simulink model "generic_IVS"  (R2024a)
settings: Solver=FixedStepDiscrete  StartTime=0.0  StopTime=inf  FixedStep=0.001  RelTol=1e-3  EnableMultiTasking=on
undefined symbols (not defined in the file or in its folder): carLengthObs, dir, ego_Accel, ego_Speed, ego_X, ego_Y, ego_YAW, goalPosTol, goalYawTol, init_CurrentLaneInfo, init_DrivingMissionInfo, init_EgoVehicle, init_HybridAStarParam, init_MapData, init_ParkingMIssionInfo, is_Optimal_Path, isPathFound, LAD, lane_Coeff, lane_Idx, lane_waypoints, lane_waypoints_Length, lookAheadDistance, maxIter, missionState, obsRadius, parking_clear, parkingDestinationPos_X, parkingDestinationPos_Y, parkingDestinationYaw, parkingMapBoundary_X_Max, parkingMapBoundary_X_Min, parkingMapBoundary_Y_Max, parkingMapBoundary_Y_Min, parkingStartPos_X, parkingStartPos_Y, R_min, reversePenalty, Route1, route1_waypoint, Route2, route2_waypoint, Route3, route3_waypoint, Route_Parking, route_parking_waypoint, steerSet, stepSize, tollgateLaneNumber, vehicleRadius, velReference, xyResolution, y_LAD, y_lookAheadDistance, yawResolution, yawWeight
libraries: CarMaker4SL x48, simulink x1
(part 4 of 4)

== matlab function generic_IVS/CarMaker/Subsystem/Final Project/Scenario 1/Subsystem8/Global Waypoints To Local Transfomer ==
  settings: sampleTime=0.05
  data: waypointList input; current_lane_info input Bus: busCurrentLaneInfo; local_waypoints_ output size=[30 2]; ego_status input Bus: busEgoVehicle
function local_waypoints_ = global_to_local_waypoints(waypointList, current_lane_info, ego_status)

    num_waypoint = 15;
    vehicle_position = [ego_status.ego_X, ego_status.ego_Y];
    head = ego_status.ego_YAW;

    sub_waypointList = current_lane_info.lane_waypoints(1:current_lane_info.lane_waypoints_Length, :);

    if isempty(waypointList) || all(waypointList(:) == 0)
        waypoints = sub_waypointList;
    else
        waypoints = single(waypointList);
    end

    dx = waypoints(:,1) - vehicle_position(1);
    dy = waypoints(:,2) - vehicle_position(2);
    dist = dx.^2 + dy.^2;

    isNotForward = (dx*cos(head) + dy*sin(head)) < 0;
    dist(isNotForward) = inf;

    [~, idx_start] = min(dist);

    idx_end = idx_start + num_waypoint - 1;
    idx_end = min(idx_end, size(waypoints,1));
    selected = waypoints(idx_start:idx_end, :);

    L = size(selected,1);
    if L < num_waypoint
        selected = [selected; repmat(selected(end,:), num_waypoint-L, 1)];
    end

    R_inv = [ cos(head),  sin(head);
             -sin(head),  cos(head) ];

    delta = bsxfun(@minus, selected, vehicle_position);
    local_waypoints_ = (R_inv * delta')';

end

== matlab function generic_IVS/CarMaker/Subsystem/Final Project/Scenario 1/Subsystem8/MATLAB Function5 ==
  settings: sampleTime=0.001
  data: current_lane_info_out output Bus: busCurrentLaneInfo; current_lane_info_in input Bus: busCurrentLaneInfo; ego_status input
function current_lane_info_out = compute_lateral(current_lane_info_in, ego_status)
    
    current_lane_info_out = current_lane_info_in;
    poly_coeff = current_lane_info_in.lane_Coeff;

    lookahead_time = 1.7;
    velocity = ego_status.ego_Speed;
    x_lookahead = velocity * lookahead_time;
    degree = length(poly_coeff) - 1;

    y_ref = single(0.0);
    for i = 0:degree
        y_ref = y_ref + poly_coeff(i+1) * x_lookahead^i;
    end

    y_LAD = y_ref;
    LAD = sqrt(x_lookahead^2 + y_LAD^2);
    % disp('---lateral Node---')
    % disp(LAD)
    % disp(y_LAD)
    
    current_lane_info_out.lookAheadDistance = LAD;
    current_lane_info_out.y_lookAheadDistance = y_LAD;
    
end

== matlab function generic_IVS/CarMaker/Subsystem/Final Project/Scenario 1/Subsystem8/MATLAB Function6 ==
  settings: sampleTime=0.05
  data: local_waypoints input; current_lane_info_out output Bus: busCurrentLaneInfo; current_lane_info_in input Bus: busCurrentLaneInfo
function current_lane_info_out = fit_polynomial_to_waypoints(local_waypoints, current_lane_info_in)
    current_lane_info_out = fit_polynomial_to_waypoints_mfile(local_waypoints, current_lane_info_in);
end

function current_lane_info_out = fit_polynomial_to_waypoints_mfile(local_waypoints, current_lane_info_in)
    
    current_lane_info_out = current_lane_info_in;
    num_degree = 3;
    N = size(local_waypoints, 1);

    x = local_waypoints(:,1);
    b = local_waypoints(:,2);

    A = zeros(N, num_degree+1);
    for i = 0:num_degree
        A(:, i+1) = x.^i;
    end
    
    poly_coeff = pinv(A) * b;
    current_lane_info_out.lane_Coeff = poly_coeff;
    
    % disp('---polyfit Node---')
    % disp(current_lane_info_out.lane_Coeff)
    
end

== matlab function generic_IVS/CarMaker/Subsystem/Final Project/Scenario 1/Subsystem9/Lateral Control/MATLAB Function7 ==
  settings: updateMethod=DISCRETE  sampleTime=0.05
  data: current_lane_info input Bus: busCurrentLaneInfo; ego_status input Bus: busEgoVehicle; delta output
function delta  = lateral_stanley_controller_(current_lane_info, ego_status)
    
    k_h = 0.8;
    k_e = 0.4;

    heading_error = atan(current_lane_info.lane_Coeff(2));
    cross_track_error = current_lane_info.y_lookAheadDistance;
    V = ego_status.ego_Speed;
    
    heading_err_term     = k_h * heading_error;
    cross_track_err_term = atan(k_e * cross_track_error / V);

    delta = (heading_err_term + cross_track_err_term);
    
    V_thresh = 1;
    if abs(V) < V_thresh
        delta = 0;
        return;
    end

end

== matlab function generic_IVS/CarMaker/Subsystem/Final Project/Scenario 1/Subsystem9/Lateral Control/MATLAB Function8 ==
  settings: updateMethod=DISCRETE  sampleTime=0.05
  data: current_lane_info input Bus: busCurrentLaneInfo; delta output
function delta  = lateral_PP_controller_(current_lane_info)
    
    L = 2.9;  %wheelbase
    LAD = current_lane_info.lookAheadDistance;
    y_LAD = current_lane_info.y_lookAheadDistance;
    heading_error = current_lane_info.lane_Coeff(2);

    if LAD == 0
        disp('LAD = 0')
        delta = single(0.0);
        return
    end

    delta = 1.05*atan( 2 * L * y_LAD / (LAD^2) );

    % disp('---PP Node---')
    % disp(LAD)
    % disp(y_LAD)
    
end

== matlab function generic_IVS/CarMaker/Subsystem/Final Project/Scenario 1/get_adj_obstacles_info ==
  settings: sampleTime=0.05
  data: ego_status input; obstacles_info input [3..10]; adj output size=[8 10]; driving_mission_info input
function adj = get_adj_obstacles_info(ego_status, obstacles_info, driving_mission_info)
    % obstacles_info   : Nx matrix or struct (each obstacle row = one vehicle)
    %                    columns assumed: [X, Y, Vx, Vy, Ax, Ay, Yaw, Yawrate]

    % disp('--------')
    % disp(obstacles_info);
    % disp('--------')
    % disp('Vehicle_position')
    % disp(vehicle_position);
    % disp('--------')

    mission_state = driving_mission_info.missionState;
    if mission_state >= 3
        adj = zeros(3, 10);
        return;
    end
    
    dist_threshhold = 30.0;
    
    ego_x = ego_status.ego_X;
    ego_y = ego_status.ego_Y;

    X = obstacles_info(:,1);
    Y = obstacles_info(:,2);

    % 거리 계산
    dx = X - ego_x;
    dy = Y - ego_y;
    dist = dx.^2 + dy.^2;

    % threshold 안에 있는 인덱스
    idx = dist < dist_threshhold^2;

    % 필터링된 장애물 정보
    adj = obstacles_info(idx, :);
    
    % disp(idx);
    % if ~isempty(adj)
    %     disp('-----')
    %     disp(adj(1, :));
    % end
end

== matlab function generic_IVS/CarMaker/Subsystem/Final Project/Scenario 1/Set Velocity Reference ==
  settings: updateMethod=DISCRETE  sampleTime=0.05
  data: ego_status input Bus: busEgoVehicle; driving_mission_info_out output Bus: busDrivingMissionInfo; driving_mission_info_in input
function driving_mission_info_out = set_velocity_ref(ego_status, driving_mission_info_in)
    
    driving_mission_info_out = driving_mission_info_in;
    target_velocity = driving_mission_info_in.velReference;
    mission_state = driving_mission_info_in.missionState;

    ego_X = ego_status.ego_X;
    ego_Y = ego_status.ego_Y;

    lane_section_idx = get_lane_section_idx(ego_X, ego_Y);

    if lane_section_idx == 0
        mission_state = uint8(4);
    end

    if lane_section_idx == 1
        target_velocity = single(55/3.6);
    elseif lane_section_idx == 3 || lane_section_idx == 6
        target_velocity = single(45/3.6);
    elseif lane_section_idx == 4
        target_velocity = single(50/3.6);
    elseif lane_section_idx == 5
        target_velocity = single(55/3.6);
    elseif lane_section_idx == 7
        target_velocity = single(50/3.6);
    
    % 직선도로
    elseif lane_section_idx == 8
        target_velocity = single(65/3.6);
    end

    
    if mission_state == 2
        target_velocity = single(30/3.6);

    elseif mission_state == 3
        target_velocity = single(20/3.6);

        if lane_section_idx == 9
            target_velocity = single(8/3.6);
        end

    elseif mission_state == 4
        target_velocity = single(0.0);
    end

    driving_mission_info_out.velReference = target_velocity;

end

function lane_section_idx = get_lane_section_idx(ego_x, ego_y)
    % 섹션 1
    section1_x = [-50.6, -50.6, -99.25, -154, -168.38, -169];
    section1_y = [27,11.6, -18.32, -46.77, -39.43,27]; 
    
    % 섹션 2
    section2_x = [-168.38, -154, -151, -166.95, -178.59, -187];
    section2_y = [-39.43, -46.77, -69.31, -85.52, -85.52, -55];
    
    % 섹션 3
    section3_x = [-178.59, -166.95, -104, -36.24, -25.19, -25.19, -178.59];
    section3_y = [-85.52, -85.52, -85.52, -110.78, -115.02, -172, -172];
    
    % 섹션 4
    section4_x = [-36.24, -25.19, 3, 4.57, 0.49, -32];
    section4_y = [-110.78, -115.02, -113, -87.46, -76, -77];
    
    % 섹션 5
    section5_x = [ 0.49, 4.57, 41, 81.24, 81.24, 33];
    section5_y = [-76, -87.46, -85, -78.92, -63.15, -55];
    
    % 섹션 6
    section6_x = [81.24, 81.24, 111.99, 124.34, 124.4];
    section6_y = [-78.92, -63.15, -38.14, -38.14, -78.92];
    
    % 섹션 7
    section7_x = [60, 60, 111.99, 124.34, 124.34];
    section7_y = [27, 11.6, -38.14, -38.14, 27];
    
    % 섹션 8 직선도로
    section8_x = [-50.6, -50.6, 60, 60];
    section8_y = [27, 11.6, 11.6, 27];
    
    % 섹션 9 주차장 입구
    section9_x = [-9.8,5.5,-9.8,5.5];
    section9_y = [11.6, 11.6,-45,-45];

    polygon_list = {
        section1_x,  section1_y;
        section2_x,  section2_y;
        section3_x,  section3_y;
        section4_x,  section4_y;
        section5_x,  section5_y;
        section6_x,  section6_y;
        section7_x,  section7_y;
        section8_x,  section8_y;
        section9_x,  section9_y;
    };
    
    lane_section_idx = uint8(0);

    for i = 1:size(polygon_list,1)
        px = polygon_list{i,1};
        py = polygon_list{i,2};

        inside = inpolygon(ego_x, ego_y, px, py);

        if inside
            lane_section_idx = uint8(i);
            return;
        end
    end

end

== matlab function generic_IVS/CarMaker/Subsystem/Final Project/Scenario 1/MATLAB Function ==
  data: parking_mission_info input Bus: busParkingMissionInfo; path output size=[20000 4]; obstacles input; param input Bus: busHybridAStarParam
function path = hybridAstar_planner(parking_mission_info, obstacles, param)
    
    persistent initialized
    persistent cached_path
    persistent cached_len

    MAX_PATH = 20000;
    if isempty(initialized)
        initialized = false;
        cached_path = zeros(MAX_PATH, 4, 'single');
        cached_len  = uint16(0);
    end

    if initialized
        path = cached_path(1:cached_len, :);
        return;
    end
    x_min = parking_mission_info.parkingMapBoundary_X_Min;
    x_max = parking_mission_info.parkingMapBoundary_X_Max;
    y_min = parking_mission_info.parkingMapBoundary_Y_Min;
    y_max = parking_mission_info.parkingMapBoundary_Y_Max;
    
    space = [x_min, x_max, y_min, y_max];

    start_X   = parking_mission_info.parkingStartPos_X;
    start_Y   = parking_mission_info.parkingStartPos_Y;
    start_YAW = 0;

    obstacles = obstacles(:,1:3);
    
    goal_X   = parking_mission_info.parkingDestinationPos_X;
    goal_Y   = parking_mission_info.parkingDestinationPos_Y;
    goal_YAW = parking_mission_info.parkingDestinationYaw;

    goal = [goal_X, goal_Y, goal_YAW];

    p = param;

    nx = single(floor((x_max - x_min) / p.xyResolution) + 1);
    ny = single(floor((y_max - y_min) / p.xyResolution) + 1);
    nyaw = single(floor(2*pi / p.yawResolution) + 1);
    
    costList    = inf(nx, ny, nyaw);
    nodeIdList  = zeros(nx, ny, nyaw);
    closedList  = false(nx, ny, nyaw);
    
    MAX_NODES   = 20000;
    MAX_OPENSET = 20000;
    MAX_CHILDREN = 6;

    nodeTemplate = struct('x',single(0), 'y',single(0), 'yaw',single(0),...
                          'g',single(0), 'h',single(0), 'f',single(0),...
                          'dir',single(1), 'parent',int32(0),...
                          'ix',single(0), 'iy',single(0), 'iyaw',single(0));

    nodes = repmat(nodeTemplate, MAX_NODES, 1);
    nodeCount = 1;

    [ix,iy,iyaw] = world2grid(start_X, start_Y, start_YAW, ...
                              x_min, y_min, p.xyResolution, p.yawResolution);

    nodes(1).x    = start_X;
    nodes(1).y    = start_Y;
    nodes(1).yaw  = wrapToPi_local(start_YAW);
    nodes(1).g    = single(0.0);
    nodes(1).h    = heuristic_cost(start_X, start_Y, start_YAW, goal, p);
    nodes(1).f    = nodes(1).g + nodes(1).h;
    nodes(1).dir  = single(1.0);
    nodes(1).parent = int32(0);
    nodes(1).ix   = ix;
    nodes(1).iy   = iy;
    nodes(1).iyaw = iyaw;

    costList(ix,iy,iyaw)   = 0;
    nodeIdList(ix,iy,iyaw) = 1;

    openSet     = zeros(MAX_OPENSET, 1, 'int32');
    openCount   = 1;
    openSet(1)  = 1;

    success = false;
    goalId  = int32(-1);

    iter = 0;
    while (openCount > 0) && (iter < p.maxIter)
        iter = iter + 1;

        bestIdx = 1;
        bestId  = openSet(1);
        bestF   = nodes(bestId).f;
        
        for i = 2:openCount
            nid = openSet(i);
            if nodes(nid).f < bestF
                bestF = nodes(nid).f;
                bestIdx = i;
                bestId  = nid;
            end
        end
        
        curId = bestId;
        openSet(bestIdx) = openSet(openCount);  % 마지막 원소와 교체
        openCount = openCount - 1;

        curNode = nodes(curId);
        if closedList(curNode.ix, curNode.iy, curNode.iyaw)
            continue;
        end
        closedList(curNode.ix, curNode.iy, curNode.iyaw) = true;

        if isGoalReached(curNode, goal, p)
            success = true;
            goalId  = int32(curId);
            break;
        end

        children = CreateNode(curNode, p);

        for k = 1:numel(children)
            child = children(k);

            if child.x < x_min || child.x > x_max || ...
               child.y < y_min || child.y > y_max
                continue;
            end

            if checkCollisionMotion(curNode, child, obstacles, space, p)
                continue;
            end

            [ix_c,iy_c,iyaw_c] = world2grid(child.x, child.y, child.yaw, ...
                                            x_min, y_min, ...
                                            p.xyResolution, p.yawResolution);

            if closedList(ix_c,iy_c,iyaw_c)
                continue;
            end

            g_new = curNode.g + child.cost;

            if g_new < costList(ix_c,iy_c,iyaw_c)
                childNode = nodeTemplate;
                childNode.x    = child.x;
                childNode.y    = child.y;
                childNode.yaw  = wrapToPi_local(child.yaw);
                childNode.g    = g_new;
                childNode.h    = heuristic_cost(childNode.x, childNode.y, childNode.yaw, goal, p);
                childNode.f    = childNode.g + childNode.h;
                childNode.dir  = child.dir;
                childNode.parent = curId;
                childNode.ix   = ix_c;
                childNode.iy   = iy_c;
                childNode.iyaw = iyaw_c;

                if nodeIdList(ix_c,iy_c,iyaw_c) == 0
                    nodeCount = nodeCount + 1;
                    if nodeCount > MAX_NODES
                        continue;
                    end

                    nodes(nodeCount) = childNode;
                    newId = nodeCount;
                else
                    newId = nodeIdList(ix_c,iy_c,iyaw_c);
                    nodes(newId) = childNode;
                end

                costList(ix_c,iy_c,iyaw_c)   = g_new;
                nodeIdList(ix_c,iy_c,iyaw_c) = newId;
                
                if openCount < MAX_OPENSET
                    openCount = openCount + 1;
                    openSet(openCount) = newId;
                else
                end

            end
        end
    end

    if ~success
        path = zeros(1,4,'single');
        if ~initialized
            visualize_hybridAstar_internal(path, obstacles, [start_X start_Y], [goal_X goal_Y], p);
            initialized = true;
        end
        disp('no path')
        return;
    end

    path = backtrackPath(nodes, goalId, MAX_NODES);
    disp('find path')
    
    valid = (path(:,1) ~= 0) | (path(:,2) ~= 0) | (path(:,3) ~= 0);
    path = path(valid, :);

    k = size(path,1);
    cached_path(1:k, :) = path;
    cached_len = uint16(k);
    initialized = true;

    visualize_hybridAstar_internal(path, obstacles, [start_X start_Y], [goal_X goal_Y], p);
end



function ang = wrapToPi_local(ang)
    ang = single(mod(ang + pi, 2*pi) - pi);
end

% 양자화 때리는거
function [ix, iy, iyaw] = world2grid(x, y, yaw, x_min, y_min, res_xy, res_yaw)
    ix = floor((x - x_min) / res_xy) + 1;
    iy = floor((y - y_min) / res_xy) + 1;
    yaw = wrapToPi_local(yaw);
    iyaw = floor((yaw + pi) / res_yaw) + 1;
end

% 도착했는지 검사
function flag = isGoalReached(node, goal, p)
    dx = goal(1) - node.x;
    dy = goal(2) - node.y;
    dist = sqrt(dx^2 + dy^2);

    dyaw = abs(wrapToPi_local(goal(3) - node.yaw));
    flag = (dist < p.goalPosTol) && (dyaw < p.goalYawTol);
end

% 자식낳기
function children = CreateNode(node, p)

    R = p.R_min;
    kappa_max = 1.0 / R;
    ds = p.stepSize;

    steeringSet = p.steerSet * kappa_max;
    dirSet = [1, -1];

    MAX_CHILDREN = 6;
    children = repmat(struct('x',single(0), 'y',single(0), 'yaw',single(0), ...
                             'dir',single(0), 'cost',single(0)), single(MAX_CHILDREN), single(1));
    childCount = 0;

    for i = 1:length(steeringSet)

        kappa = steeringSet(i);
        for d = 1:length(dirSet)
            dir = dirSet(d);
            s   = dir * ds;

            [xn, yn, yawn] = BicycleKinematic(node.x, node.y, node.yaw, kappa, s);

            % cost: 경로 길이 + 후진 패널티
            cost = abs(ds);
            if dir < 0
                cost = cost * p.reversePenalty;
            end

            childCount = childCount + 1;
            children(childCount).x    = xn;
            children(childCount).y    = yn;
            children(childCount).yaw  = yawn;
            children(childCount).dir  = single(dir);
            children(childCount).cost = cost;
        end
    end
end

% Bicycle 모델
function [x_new, y_new, yaw_new] = BicycleKinematic(x, y, yaw, kappa, s)
    if abs(kappa) < 1e-6

        x_new   = x + s * cos(yaw);
        y_new   = y + s * sin(yaw);
        yaw_new = yaw;
    else

        R = 1.0 / kappa;
        yaw_new = yaw + kappa * s;
        x_new = x + R * (sin(yaw_new) - sin(yaw));
        y_new = y - R * (cos(yaw_new) - cos(yaw));
    end
    yaw_new = wrapToPi_local(yaw_new);
end

% 중간 샘플 몇 개 찍어서 충돌 체크 할거임
function flag = checkCollisionMotion(n1, n2, obstacles, space, p)
    
    nSamples = 5;
    flag = false;

    kappa_est = curvatureFromNodes(n1, n2, p);

    for i = 0:nSamples
        t  = i / nSamples;
        s  = t * p.stepSize * sign(n2.dir); % 방향 고려
        [x_s, y_s, ~] = BicycleKinematic(n1.x, n1.y, n1.yaw, ...
                                           kappa_est, s);

        if checkCollisionPoint(x_s, y_s, obstacles, space, p)
            flag = true;
            return;
        end
    end
end

function flag = checkCollisionPoint(x, y, obstacles, space, p)
    % World boundary
    if x < space(1) || x > space(2) || ...
       y < space(3) || y > space(4)
        flag = true;
        return;
    end

    % 장애물: 뒷대가리 기준 + heading → 차량 길이 따라 원 2개 배치
    L = p.carLengthObs;
    
    d1 = L * 0.3;    % 뒤쪽 쪽
    d2 = L * 0.8;    % 앞쪽 쪽

    effR2 = (p.obsRadius + p.vehicleRadius)^2;

    for i = 1:size(obstacles,1)
        xr = obstacles(i,1);
        yr = obstacles(i,2);
        hdg = obstacles(i,3);

        % 두 개 서클의 중심
        x1 = xr + d1*cos(hdg);
        y1 = yr + d1*sin(hdg);
        x2 = xr + d2*cos(hdg);
        y2 = yr + d2*sin(hdg);

        dx1 = x - x1; dy1 = y - y1;
        dx2 = x - x2; dy2 = y - y2;

        if (dx1*dx1 + dy1*dy1 < effR2) || (dx2*dx2 + dy2*dy2 < effR2)
            flag = true;
            return;
        end
    end

    flag = false;
end

function kappa = curvatureFromNodes(n1, n2, p)
    % n1→n2 κ 추정 (대충 yaw 변화로 계산)
    ds = p.stepSize;
    dyaw = wrapToPi_local(n2.yaw - n1.yaw);
    if abs(ds) < 1e-6
        kappa = single(0);
    else
        kappa = single(dyaw / (ds * sign(n2.dir)));
    end
end

function h = heuristic_cost(x, y, yaw, goal, p)
    dx = goal(1) - x;
    dy = goal(2) - y;
    dist = sqrt(dx^2 + dy^2);

    dyaw = abs(wrapToPi_local(goal(3) - yaw));
    h = dist + p.yawWeight * dyaw;
end

function path = backtrackPath(nodes, goalId, MAX_PATH)
    path = zeros(MAX_PATH, 4, 'single');

    idx = goalId;
    k = 0;
    
    % 뒤에서부터 채우고 뒤집음
    while (idx ~= 0) && (k < MAX_PATH)
        n = nodes(idx);
        k = k + 1;
        path(k, :) = [n.x, n.y, n.yaw, n.dir];
        idx = n.parent;
    end

    if k > 1
        % start→goal 순서로 뒤집기
        path(1:k, :) = flipud(path(1:k, :));
    end
end

% 시각화 (한번만 함)
function visualize_hybridAstar_internal(path, obstacles, startXY, goalXY, p)

    figure; hold on; axis equal; grid on;
    xlabel('X'); ylabel('Y');
    title('Hybrid A* Path');

    for i = 1:size(obstacles,1)
        drawObstacleCarDual(obstacles(i,1), obstacles(i,2), obstacles(i,3), p);
    end

    % Start & Goal
    plot(startXY(1), startXY(2), 'go', 'MarkerFaceColor','g','MarkerSize',10);
    plot(goalXY(1),  goalXY(2),  'ro', 'MarkerFaceColor','r','MarkerSize',10);

    % Path
    xs = path(:,1); ys = path(:,2); dirs = path(:,4);
    valid = xs ~= 0;
    xs = xs(valid); ys = ys(valid); dirs = dirs(valid);

    for i = 1:length(xs)-1
        if dirs(i) > 0
            plot(xs(i:i+1), ys(i:i+1), 'b-', 'LineWidth', 2);
        else
            plot(xs(i:i+1), ys(i:i+1), 'r-', 'LineWidth', 2);
        end
    end

    hold off;
end


function h = drawCircle(x, y, r, color)
    th = linspace(0, 2*pi, 40);
    xc = x + r*cos(th);
    yc = y + r*sin(th);
    h = fill(xc, yc, color, 'FaceAlpha', 0.3, 'EdgeColor', color);
end

function drawObstacleCarDual(xr, yr, hdg_deg, p)
    L   = p.carLengthObs;
    hdg = hdg_deg;

    d1 = L * 0.3;
    d2 = L * 0.8;

    x1 = xr + d1*cos(hdg);
    y1 = yr + d1*sin(hdg);
    x2 = xr + d2*cos(hdg);
    y2 = yr + d2*sin(hdg);

    drawCircle(x1, y1, p.obsRadius, [0.7 0.2 0.2]);
    drawCircle(x2, y2, p.obsRadius, [0.7 0.2 0.2]);
end

== matlab function generic_IVS/CarMaker/Subsystem/Final Project/Scenario 1/Global Waypoints To Local Transfomer ==
  settings: sampleTime=0.05
  data: mission_state input; parking_mission_info_in input Bus: busParkingMissionInfo; parking_mission_info_out output Bus: busParkingMissionInfo; waypoints input; ego_status input Bus: busEgoVehicle
function parking_mission_info_out  = global_to_local_path_manager(mission_state, parking_mission_info_in, waypoints, ego_status)
    
    parking_mission_info_out = parking_mission_info_in;
    
    if mission_state ~= 4
        return;
    end

    goalX = parking_mission_info_in.parkingDestinationPos_X;
    goalY = parking_mission_info_in.parkingDestinationPos_Y;
    ego_X = ego_status.ego_X;
    ego_Y = ego_status.ego_Y;

    dx_goal = ego_X - goalX;
    dy_goal = ego_Y - goalY;
    dist_goal = sqrt(dx_goal^2 + dy_goal^2);

    if dist_goal < 1.0
        parking_mission_info_out.parking_clear = uint8(1);
        parking_mission_info_out.LAD = single(0.01);
        parking_mission_info_out.y_LAD = single(0.0);
        disp("Parking!")
        return;
    end
    
    if size(waypoints,1) == 1 && (max(abs(waypoints(:))) == 0)
        parking_mission_info_out.isPathFound = uint8(0);
        parking_mission_info_out.LAD = single(0.0);
        parking_mission_info_out.y_LAD = single(0.0);
        return;
    else
        parking_mission_info_out.isPathFound = uint8(1);
    end
    num_waypoint = 5;

    vehicle_position = [ego_X, ego_Y];
    head = ego_status.ego_YAW;

    dx = waypoints(:,1) - vehicle_position(1);
    dy = waypoints(:,2) - vehicle_position(2);
    dist = dx.^2 + dy.^2;

    % isNotForward = (dx*cos(head) + dy*sin(head)) < 0;
    % dist(isNotForward) = inf;

    [minDist, idx_start] = min(dist);
    
    % disp('---minDist---')
    % disp(minDist)
    % if minDist > 3.0
    %     parking_mission_info_out.LAD = single(0.0);
    %     parking_mission_info_out.y_LAD = single(0.0);
    %     parking_mission_info_out.dir = int8(-1);
    %    return;
    % end

    idx_end = idx_start + num_waypoint - 1;
    idx_end = min(idx_end, size(waypoints,1));
    selected = waypoints(idx_start:idx_end, :);

    L = size(selected,1);
    if L < num_waypoint
        selected = [selected; repmat(selected(end,:), num_waypoint-L, 1)];
    end

    R_inv = [ cos(head),  sin(head);
             -sin(head),  cos(head) ];
    
    selected_xy = selected(:,1:2);
    delta = bsxfun(@minus, selected_xy, vehicle_position);
    local_waypoints_ = (R_inv * delta')';

    poly_coeff  = fit_polynomial_to_waypoints_mfile(local_waypoints_);
    [y_LAD, LAD] = compute_lateral(poly_coeff);
    dir = int8(waypoints(idx_start,4));

    % disp(size(waypoints(:,1)))
    % disp(idx_start)
    % disp(waypoints(idx_start, :))
    
    parking_mission_info_out.LAD = LAD;
    parking_mission_info_out.y_LAD = y_LAD;
    parking_mission_info_out.dir = dir;

end

function  poly_coeff  = fit_polynomial_to_waypoints_mfile(local_waypoints)

    num_degree = 3;
    N = size(local_waypoints, 1);

    x = local_waypoints(:,1);
    b = local_waypoints(:,2);

    A = zeros(N, num_degree+1);
    for i = 0:num_degree
        A(:, i+1) = x.^i;
    end
    
    poly_coeff = pinv(A) * b;
    
end

function [y_LAD, LAD] = compute_lateral(poly_coeff)

    x_lookahead = 2.9 + 0.6;
    degree = length(poly_coeff) - 1;

    y_ref = single(0.0);
    for i = 0:degree
        y_ref = y_ref + poly_coeff(i+1) * x_lookahead^i;
    end

    y_LAD = single(y_ref);
    LAD = single(sqrt(x_lookahead^2 + y_LAD^2));
    
end

== stateflow chart generic_IVS/CarMaker/Subsystem/Final Project/Scenario 1/Subsystem7/Chart3 ==
  state driving
    mission=1;
  state tollgate
    mission=2;
  state parking_entry
    mission=3;
  state parking
    mission=4;
  (default) -> driving
  driving -> tollgate [order 1] : [flag_2==1]
  tollgate -> driving : [flag_2==0]
  driving -> parking_entry [order 2] : [flag_3==1]
  parking_entry -> parking : [flag_4==1]
  data: flag_2 input; flag_3 input; mission output; flag_4 input

== matlab function generic_IVS/CarMaker/Subsystem/Final Project/Scenario 1/Subsystem6/MATLAB Function9 ==
  data: ego_status input; tollgate_pass_mode output
function tollgate_pass_mode = check_tollgate(ego_status)
% CHECK_TOLLGATE_ZONE: 에고 차량이 톨게이트 영역 내에 있는지 확인하여 플래그를 반환합니다.
%
% 입력:
%   ego_global_x: 에고 차량의 현재 글로벌 X 좌표 (float)
%   ego_global_y: 에고 차량의 현재 글로벌 Y 좌표 (float)


% 출력:
%   tollgate_pass_mode: 0 (영역 밖) 또는 1 (영역 내) (int)

    % 1. 톨게이트 영역 경계 정의
    min_x = -190;
    max_x = -90;
    min_y = -165;
    max_y = -86;
    
    ego_global_x = ego_status.ego_X;
    ego_global_y = ego_status.ego_Y;

    % 2. 플래그 설정 로직
    if (ego_global_x >= min_x && ego_global_x <= max_x) && ...
       (ego_global_y >= min_y && ego_global_y <= max_y)
        % 에고 차량이 영역 내에 있는지 확인
        tollgate_pass_mode = 1;
    else
        % 그렇지 않을 경우 (영역 밖)
        tollgate_pass_mode = 0;
    end
    
    %
end

== matlab function generic_IVS/CarMaker/Subsystem/Final Project/Scenario 1/Subsystem6/MATLAB Function10 ==
  data: ego_status input; parking_entry_mode output; IS_FRONT input
function parking_entry_mode = check_parking_entry(ego_status, IS_FRONT)
    % Simulink MATLAB Function 블록용 주차 진입 플래그 로직 (수정됨)
    
    % 영구 변수(Persistent Variables) 선언
    persistent parking_entry_flag Pass_Count In_Boundary_Prev TARGET_PASS_COUNT IsInitialized
    parking_entry_mode = uint8(0);

    Ego_Global_X = ego_status.ego_X;
    Ego_Global_Y = ego_status.ego_Y;
    % BOUNDARY 변수 정의 (시뮬레이션 환경에 맞게 조정 필요)
    BOUND_X_MIN = -108;
    BOUND_X_MAX = -95;
    BOUND_Y_MIN = -3;
    BOUND_Y_MAX = 17;
    
    % X_MAX = -95;
    % X_MIN = -108;
    % Y_MIN = 3;
    % Y_MAX = 17;
    
    % --- 1. 초기화 (시뮬레이션 시작 시 단 한 번 실행) ---
    if isempty(IsInitialized)
        
        % A. IS_FRONT 값에 기반하여 Target_Pass_Count 설정
        if IS_FRONT == 1
            % 앞 시작: 1번째 진입 시 플래그 활성화
            TARGET_PASS_COUNT = uint8(1); 
        else
            % 뒤 시작: 2번째 진입 시 플래그 활성화
            TARGET_PASS_COUNT = uint8(2);
        end
    
        % 초기 상태 설정 (타입 캐스팅 적용)
        parking_entry_flag = uint8(0);
        Pass_Count = uint8(0);         
        In_Boundary_Prev = false; 
        IsInitialized = true;
    end
    
    % --- 2. 실시간 업데이트 (매 스텝마다 실행) ---
    
    % 1. 이미 플래그가 1이면 더 이상 계산할 필요 없음
    if parking_entry_flag == 1
        parking_entry_flag = uint8(parking_entry_flag);
        return;
    end
    
    % 2. 현재 바운더리 상태 확인
    In_Boundary_Curr = (Ego_Global_X >= BOUND_X_MIN && Ego_Global_X <= BOUND_X_MAX && ...
                        Ego_Global_Y >= BOUND_Y_MIN && Ego_Global_Y <= BOUND_Y_MAX);
    
    % 3. 통과 횟수 업데이트 (밖 -> 안 진입 감지)
    if In_Boundary_Curr && ~In_Boundary_Prev
        Pass_Count = Pass_Count + uint8(1);
    end
    
    % 4. 플래그 활성화 조건 확인
    % Pass_Count가 목표 횟수와 같아지는 순간 플래그 활성화
    if Pass_Count == TARGET_PASS_COUNT
        parking_entry_flag = uint8(1);
    end
    
    % 5. 다음 스텝을 위한 상태 저장
    In_Boundary_Prev = In_Boundary_Curr;
    
    parking_entry_mode = uint8(parking_entry_flag); 

end

== matlab function generic_IVS/CarMaker/Subsystem/Final Project/Scenario 1/Subsystem6/MATLAB Function11 ==
  data: ego_status input; parking_mode output
function parking_mode = check_parking_zone(ego_status)


% 입력:
%   ego_global_x: 에고 차량의 현재 글로벌 X 좌표 (float)
%   ego_global_y: 에고 차량의 현재 글로벌 Y 좌표 (float)
%   tollgate_zone_x_limits: 톨게이트 영역의 X축 경계 [min_x, max_x]
%   tollgate_zone_y_limits: 톨게이트 영역의 Y축 경계 [min_y, max_y]
%
% 출력:
%   주차장 모드 0 (영역 밖) 또는 1 (영역 내) (int)
    
    parking_mode = 0;

    ego_global_X = ego_status.ego_X;
    ego_global_Y = ego_status.ego_Y;
    % 1. 주차장 영역 -> 여기로 들어오면 parking
    min_x = -2.5;
    max_x = 5.5;
    min_y = -38.5;
    max_y = -25.5;

    % 2. 플래그 설정 로직
    if (ego_global_X >= min_x && ego_global_X <= max_x) && ...
       (ego_global_Y >= min_y && ego_global_Y <= max_y)
        
        parking_mode = 1;
    end
    
end

== matlab function generic_IVS/CarMaker/Subsystem/Final Project/Scenario 1/Subsystem11/Lateral Control/MATLAB Function8 ==
  settings: updateMethod=DISCRETE  sampleTime=0.01
  data: parking_mission_info input Bus: busParkingMissionInfo; delta output; ego_status input
function delta  = lateral_PP_controller_(parking_mission_info, ego_status)
    
    L = 2.9;  %wheelbase
    LAD = parking_mission_info.LAD;
    y_LAD = parking_mission_info.y_LAD;

    if LAD == 0
        disp('LAD = 0')
        delta = single(0.0);
        return
    end

    delta = 0.9*atan( 2 * L * y_LAD / (LAD^2) );
    % if parking_mission_info.dir < 0
    %     delta = -delta;
    % end

    % disp('---PP Node---')
    % disp(LAD)
    % disp(y_LAD)
    
end

== stateflow chart generic_IVS/CarMaker/Subsystem/Day3/Chart ==
  (default) -> (junction 1)
  (junction 1) -> (junction 3) [order 1] : [i<99]
      | {i = i + 1;}
  (junction 1) -> (junction 7) [order 2] : {i=0;}
  (junction 3) -> (junction 5)
  (junction 5) -> (junction 7)
  (junction 7) -> (junction 10)
  (junction 10) -> (junction 12) [order 1] : [rem(i,50) == 0]
      | {do_Logic;}
  (junction 10) -> (junction 18) [order 2]
  (junction 12) -> (junction 16)
  (junction 16) -> (junction 18)
  (junction 18) -> (junction 21)
  data: i local =0
  events: do_Logic output FUNCTION_CALL_EVENT
